simulink model "Logical_Ventilation"  (R2023b)
settings: Solver=VariableStepAuto  StartTime=0.0  StopTime=60  RelTol=1e-3
PostLoadFcn:
  | load data\rel_humidity.mat;
  | load data\rel_humidity_heatedwire.mat;
  | load data\rel_humidityInput.mat;
libraries: slident x2, slpidlib x2
settings Model: DataDictionary=Logical_Ventilation_dict.sldd  Creator=ppatel  LastModifiedBy=ppatel

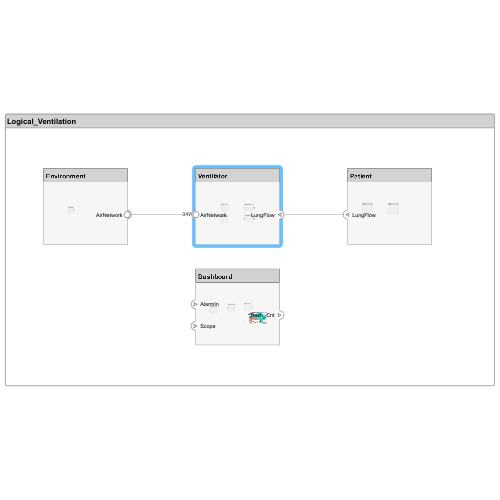
[thumbnail: Simulink's stored preview of the top-level diagram]
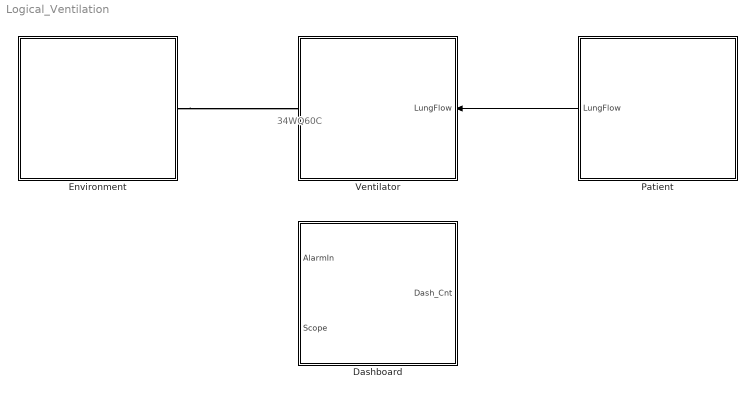
== system Logical_Ventilation ==
  note: 34WQ60C
  Dashboard : Subsystem
      settings: PortSchema="{\"entries\":[{\"content\":{\"headerSize\":26,\"margin\":15,\"minimumSpacing\":25,\"sides\":[{\"content\":{\"connectorIds\":[\"In1\",\"In2\"]},\"type\":\"ConnectorPlacement.EquallySpacedRectSide\",\"uuid\":\"30d5a539-2c7a-40a6-b159-872080309fb0\"},{\"content\":{\"connectorIds\":[\"Out1\"],\"side\":\"RIGHT\"},\"type\":\"ConnectorPlacement.EquallySpacedRectSide\",\"uuid\":\"9c23b845-c6d3-461f-9717-3c81fce4740e\"},{\"content\":{\"side\":\"TOP\"},\"type\":\"ConnectorPlacement.EquallySpacedRectSide\",\"uuid\":\"23e2f61e-2083-47d3-9d3a-aca5cd4f1fc6\"}]},\"type\":\"ConnectorPlacement.EquallySpacedConnector\",\"uuid\":\"a2e9d942-417e-49d1-8834-66036fdf29fe\"}],\"packageUris\":[\"http://schema.mathworks.com/mf0/Connector/R2020b\"],\"version\":\"1.0\"}"
  Environment : Subsystem
      settings: PortSchema="{\"entries\":[{\"content\":{\"headerSize\":26,\"margin\":15,\"minimumSpacing\":25,\"sides\":[{\"content\":{},\"type\":\"ConnectorPlacement.EquallySpacedRectSide\",\"uuid\":\"30d5a539-2c7a-40a6-b159-872080309fb0\"},{\"content\":{\"connectorIds\":[\"RConn1\"],\"side\":\"RIGHT\"},\"type\":\"ConnectorPlacement.EquallySpacedRectSide\",\"uuid\":\"9c23b845-c6d3-461f-9717-3c81fce4740e\"},{\"content\":{\"side\":\"TOP\"},\"type\":\"ConnectorPlacement.EquallySpacedRectSide\",\"uuid\":\"23e2f61e-2083-47d3-9d3a-aca5cd4f1fc6\"}]},\"type\":\"ConnectorPlacement.EquallySpacedConnector\",\"uuid\":\"a2e9d942-417e-49d1-8834-66036fdf29fe\"}],\"packageUris\":[\"http://schema.mathworks.com/mf0/Connector/R2020b\"],\"version\":\"1.0\"}"
  Patient : Subsystem
      settings: PortSchema="{\"entries\":[{\"content\":{\"headerSize\":26,\"margin\":15,\"minimumSpacing\":25,\"sides\":[{\"content\":{\"connectorIds\":[\"Out1\"]},\"type\":\"ConnectorPlacement.EquallySpacedRectSide\",\"uuid\":\"30d5a539-2c7a-40a6-b159-872080309fb0\"},{\"content\":{\"side\":\"RIGHT\"},\"type\":\"ConnectorPlacement.EquallySpacedRectSide\",\"uuid\":\"9c23b845-c6d3-461f-9717-3c81fce4740e\"},{\"content\":{\"side\":\"TOP\"},\"type\":\"ConnectorPlacement.EquallySpacedRectSide\",\"uuid\":\"23e2f61e-2083-47d3-9d3a-aca5cd4f1fc6\"}]},\"type\":\"ConnectorPlacement.EquallySpacedConnector\",\"uuid\":\"a2e9d942-417e-49d1-8834-66036fdf29fe\"}],\"packageUris\":[\"http://schema.mathworks.com/mf0/Connector/R2020b\"],\"version\":\"1.0\"}"
  Ventilator : Subsystem
      settings: PortSchema="{\"entries\":[{\"content\":{\"headerSize\":26,\"margin\":15,\"minimumSpacing\":25,\"sides\":[{\"content\":{\"connectorIds\":[\"RConn1\"]},\"type\":\"ConnectorPlacement.EquallySpacedRectSide\",\"uuid\":\"30d5a539-2c7a-40a6-b159-872080309fb0\"},{\"content\":{\"connectorIds\":[\"In1\"],\"side\":\"RIGHT\"},\"type\":\"ConnectorPlacement.EquallySpacedRectSide\",\"uuid\":\"9c23b845-c6d3-461f-9717-3c81fce4740e\"},{\"content\":{\"side\":\"TOP\"},\"type\":\"ConnectorPlacement.EquallySpacedRectSide\",\"uuid\":\"23e2f61e-2083-47d3-9d3a-aca5cd4f1fc6\"}]},\"type\":\"ConnectorPlacement.EquallySpacedConnector\",\"uuid\":\"a2e9d942-417e-49d1-8834-66036fdf29fe\"}],\"packageUris\":[\"http://schema.mathworks.com/mf0/Connector/R2020b\"],\"version\":\"1.0\"}"
  wires:
  Patient/1(LungFlow) -> Ventilator/1(LungFlow)
  connections:
  Environment/RConn1 -- Ventilator/RConn1

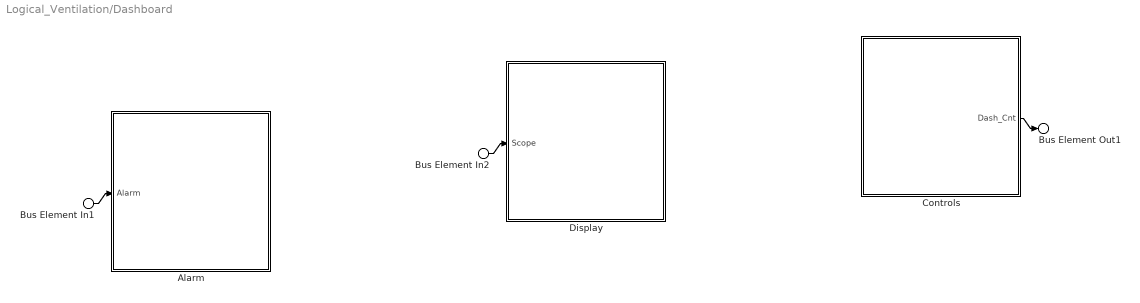
== system Logical_Ventilation/Dashboard ==
  Bus Element In1 : Inport  PortName=AlarmIn
  Bus Element In2 : Inport  Port=2  PortName=Scope
  Alarm : Subsystem
      settings: PortSchema="{\"entries\":[{\"content\":{\"headerSize\":26,\"margin\":15,\"minimumSpacing\":25,\"sides\":[{\"content\":{\"connectorIds\":[\"In1\"]},\"type\":\"ConnectorPlacement.EquallySpacedRectSide\",\"uuid\":\"30d5a539-2c7a-40a6-b159-872080309fb0\"},{\"content\":{\"side\":\"RIGHT\"},\"type\":\"ConnectorPlacement.EquallySpacedRectSide\",\"uuid\":\"9c23b845-c6d3-461f-9717-3c81fce4740e\"},{\"content\":{\"side\":\"TOP\"},\"type\":\"ConnectorPlacement.EquallySpacedRectSide\",\"uuid\":\"23e2f61e-2083-47d3-9d3a-aca5cd4f1fc6\"}]},\"type\":\"ConnectorPlacement.EquallySpacedConnector\",\"uuid\":\"a2e9d942-417e-49d1-8834-66036fdf29fe\"}],\"packageUris\":[\"http://schema.mathworks.com/mf0/Connector/R2020b\"],\"version\":\"1.0\"}"
  Controls : Subsystem
      settings: PortSchema="{\"entries\":[{\"content\":{\"headerSize\":26,\"margin\":15,\"minimumSpacing\":25,\"sides\":[{\"content\":{},\"type\":\"ConnectorPlacement.EquallySpacedRectSide\",\"uuid\":\"30d5a539-2c7a-40a6-b159-872080309fb0\"},{\"content\":{\"connectorIds\":[\"Out1\"],\"side\":\"RIGHT\"},\"type\":\"ConnectorPlacement.EquallySpacedRectSide\",\"uuid\":\"9c23b845-c6d3-461f-9717-3c81fce4740e\"},{\"content\":{\"side\":\"TOP\"},\"type\":\"ConnectorPlacement.EquallySpacedRectSide\",\"uuid\":\"23e2f61e-2083-47d3-9d3a-aca5cd4f1fc6\"}]},\"type\":\"ConnectorPlacement.EquallySpacedConnector\",\"uuid\":\"a2e9d942-417e-49d1-8834-66036fdf29fe\"}],\"packageUris\":[\"http://schema.mathworks.com/mf0/Connector/R2020b\"],\"version\":\"1.0\"}"
  Display : Subsystem
      settings: PortSchema="{\"entries\":[{\"content\":{\"headerSize\":26,\"margin\":15,\"minimumSpacing\":25,\"sides\":[{\"content\":{\"connectorIds\":[\"In1\"]},\"type\":\"ConnectorPlacement.EquallySpacedRectSide\",\"uuid\":\"30d5a539-2c7a-40a6-b159-872080309fb0\"},{\"content\":{\"side\":\"RIGHT\"},\"type\":\"ConnectorPlacement.EquallySpacedRectSide\",\"uuid\":\"9c23b845-c6d3-461f-9717-3c81fce4740e\"},{\"content\":{\"side\":\"TOP\"},\"type\":\"ConnectorPlacement.EquallySpacedRectSide\",\"uuid\":\"23e2f61e-2083-47d3-9d3a-aca5cd4f1fc6\"}]},\"type\":\"ConnectorPlacement.EquallySpacedConnector\",\"uuid\":\"a2e9d942-417e-49d1-8834-66036fdf29fe\"}],\"packageUris\":[\"http://schema.mathworks.com/mf0/Connector/R2020b\"],\"version\":\"1.0\"}"
  Bus Element Out1 : Outport  PortName=Dash_Cnt
  wires:
  Controls/1(Dash_Cnt) -> Bus Element Out1/1
  Bus Element In2/1 -> Display/1(Scope)
  Bus Element In1/1 -> Alarm/1(Alarm)

== system Logical_Ventilation/Environment ==
  Source_Sink_Air : Subsystem
      settings: PortSchema="{\"entries\":[{\"content\":{\"headerSize\":26,\"margin\":15,\"minimumSpacing\":25,\"sides\":[{\"content\":{},\"type\":\"ConnectorPlacement.EquallySpacedRectSide\",\"uuid\":\"30d5a539-2c7a-40a6-b159-872080309fb0\"},{\"content\":{\"connectorIds\":[\"RConn1\"],\"side\":\"RIGHT\"},\"type\":\"ConnectorPlacement.EquallySpacedRectSide\",\"uuid\":\"9c23b845-c6d3-461f-9717-3c81fce4740e\"},{\"content\":{\"side\":\"TOP\"},\"type\":\"ConnectorPlacement.EquallySpacedRectSide\",\"uuid\":\"23e2f61e-2083-47d3-9d3a-aca5cd4f1fc6\"}]},\"type\":\"ConnectorPlacement.EquallySpacedConnector\",\"uuid\":\"a2e9d942-417e-49d1-8834-66036fdf29fe\"}],\"packageUris\":[\"http://schema.mathworks.com/mf0/Connector/R2020b\"],\"version\":\"1.0\"}"
  AirNetwork : PMIOPort  Side=Right  ConnectionType=Bus: AirSupply
  connections:
  Source_Sink_Air/RConn1 -- AirNetwork/RConn1

== system Logical_Ventilation/Patient ==
  Lung : Subsystem
      settings: PortSchema="{\"entries\":[{\"content\":{\"headerSize\":26,\"margin\":15,\"minimumSpacing\":25,\"sides\":[{\"content\":{},\"type\":\"ConnectorPlacement.EquallySpacedRectSide\",\"uuid\":\"30d5a539-2c7a-40a6-b159-872080309fb0\"},{\"content\":{\"side\":\"RIGHT\"},\"type\":\"ConnectorPlacement.EquallySpacedRectSide\",\"uuid\":\"9c23b845-c6d3-461f-9717-3c81fce4740e\"},{\"content\":{\"side\":\"TOP\"},\"type\":\"ConnectorPlacement.EquallySpacedRectSide\",\"uuid\":\"23e2f61e-2083-47d3-9d3a-aca5cd4f1fc6\"}]},\"type\":\"ConnectorPlacement.EquallySpacedConnector\",\"uuid\":\"a2e9d942-417e-49d1-8834-66036fdf29fe\"}],\"packageUris\":[\"http://schema.mathworks.com/mf0/Connector/R2020b\"],\"version\":\"1.0\"}"
  Mask : Subsystem
      settings: PortSchema="{\"entries\":[{\"content\":{\"headerSize\":26,\"margin\":15,\"minimumSpacing\":25,\"sides\":[{\"content\":{},\"type\":\"ConnectorPlacement.EquallySpacedRectSide\",\"uuid\":\"30d5a539-2c7a-40a6-b159-872080309fb0\"},{\"content\":{\"side\":\"RIGHT\"},\"type\":\"ConnectorPlacement.EquallySpacedRectSide\",\"uuid\":\"9c23b845-c6d3-461f-9717-3c81fce4740e\"},{\"content\":{\"side\":\"TOP\"},\"type\":\"ConnectorPlacement.EquallySpacedRectSide\",\"uuid\":\"23e2f61e-2083-47d3-9d3a-aca5cd4f1fc6\"}]},\"type\":\"ConnectorPlacement.EquallySpacedConnector\",\"uuid\":\"a2e9d942-417e-49d1-8834-66036fdf29fe\"}],\"packageUris\":[\"http://schema.mathworks.com/mf0/Connector/R2020b\"],\"version\":\"1.0\"}"
  Bus Element Out1 : Outport  PortName=LungFlow

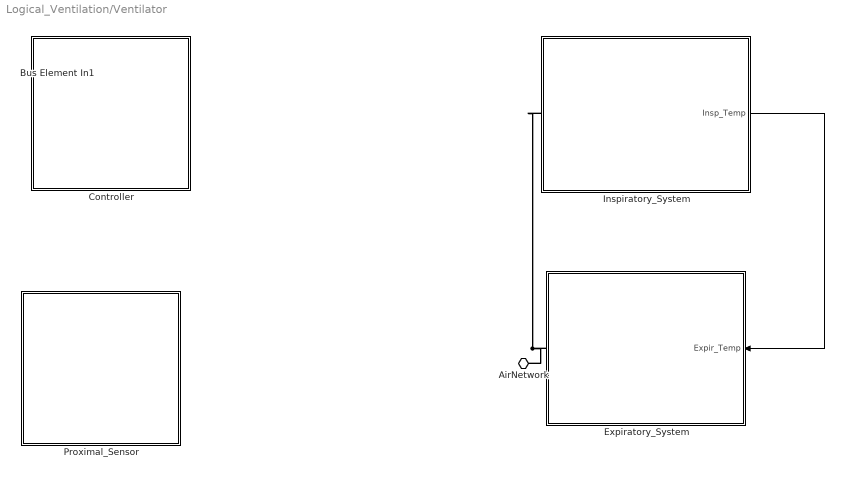
== system Logical_Ventilation/Ventilator ==
  Bus Element In1 : Inport  PortName=LungFlow
  Controller : Subsystem
      settings: PortSchema="{\"entries\":[{\"content\":{\"headerSize\":26,\"margin\":15,\"minimumSpacing\":25,\"sides\":[{\"content\":{},\"type\":\"ConnectorPlacement.EquallySpacedRectSide\",\"uuid\":\"30d5a539-2c7a-40a6-b159-872080309fb0\"},{\"content\":{\"side\":\"RIGHT\"},\"type\":\"ConnectorPlacement.EquallySpacedRectSide\",\"uuid\":\"9c23b845-c6d3-461f-9717-3c81fce4740e\"},{\"content\":{\"side\":\"TOP\"},\"type\":\"ConnectorPlacement.EquallySpacedRectSide\",\"uuid\":\"23e2f61e-2083-47d3-9d3a-aca5cd4f1fc6\"}]},\"type\":\"ConnectorPlacement.EquallySpacedConnector\",\"uuid\":\"a2e9d942-417e-49d1-8834-66036fdf29fe\"}],\"packageUris\":[\"http://schema.mathworks.com/mf0/Connector/R2020b\"],\"version\":\"1.0\"}"
  Expiratory_System : Subsystem
      settings: PortSchema="{\"entries\":[{\"content\":{\"headerSize\":26,\"margin\":15,\"minimumSpacing\":25,\"sides\":[{\"content\":{\"connectorIds\":[\"LConn1\"]},\"type\":\"ConnectorPlacement.EquallySpacedRectSide\",\"uuid\":\"30d5a539-2c7a-40a6-b159-872080309fb0\"},{\"content\":{\"connectorIds\":[\"In1\"],\"side\":\"RIGHT\"},\"type\":\"ConnectorPlacement.EquallySpacedRectSide\",\"uuid\":\"9c23b845-c6d3-461f-9717-3c81fce4740e\"},{\"content\":{\"side\":\"TOP\"},\"type\":\"ConnectorPlacement.EquallySpacedRectSide\",\"uuid\":\"23e2f61e-2083-47d3-9d3a-aca5cd4f1fc6\"}]},\"type\":\"ConnectorPlacement.EquallySpacedConnector\",\"uuid\":\"a2e9d942-417e-49d1-8834-66036fdf29fe\"}],\"packageUris\":[\"http://schema.mathworks.com/mf0/Connector/R2020b\"],\"version\":\"1.0\"}"
  Inspiratory_System : Subsystem
      settings: PortSchema="{\"entries\":[{\"content\":{\"headerSize\":26,\"margin\":15,\"minimumSpacing\":25,\"sides\":[{\"content\":{\"connectorIds\":[\"LConn1\"]},\"type\":\"ConnectorPlacement.EquallySpacedRectSide\",\"uuid\":\"30d5a539-2c7a-40a6-b159-872080309fb0\"},{\"content\":{\"connectorIds\":[\"Out1\"],\"side\":\"RIGHT\"},\"type\":\"ConnectorPlacement.EquallySpacedRectSide\",\"uuid\":\"9c23b845-c6d3-461f-9717-3c81fce4740e\"},{\"content\":{\"side\":\"TOP\"},\"type\":\"ConnectorPlacement.EquallySpacedRectSide\",\"uuid\":\"23e2f61e-2083-47d3-9d3a-aca5cd4f1fc6\"}]},\"type\":\"ConnectorPlacement.EquallySpacedConnector\",\"uuid\":\"a2e9d942-417e-49d1-8834-66036fdf29fe\"}],\"packageUris\":[\"http://schema.mathworks.com/mf0/Connector/R2020b\"],\"version\":\"1.0\"}"
  Proximal_Sensor : Subsystem
      settings: PortSchema="{\"entries\":[{\"content\":{\"headerSize\":26,\"margin\":15,\"minimumSpacing\":25,\"sides\":[{\"content\":{},\"type\":\"ConnectorPlacement.EquallySpacedRectSide\",\"uuid\":\"30d5a539-2c7a-40a6-b159-872080309fb0\"},{\"content\":{\"side\":\"RIGHT\"},\"type\":\"ConnectorPlacement.EquallySpacedRectSide\",\"uuid\":\"9c23b845-c6d3-461f-9717-3c81fce4740e\"},{\"content\":{\"side\":\"TOP\"},\"type\":\"ConnectorPlacement.EquallySpacedRectSide\",\"uuid\":\"23e2f61e-2083-47d3-9d3a-aca5cd4f1fc6\"}]},\"type\":\"ConnectorPlacement.EquallySpacedConnector\",\"uuid\":\"a2e9d942-417e-49d1-8834-66036fdf29fe\"}],\"packageUris\":[\"http://schema.mathworks.com/mf0/Connector/R2020b\"],\"version\":\"1.0\"}"
  AirNetwork : PMIOPort  Side=Right  ConnectionType=Bus: AirSupply
  wires:
  Inspiratory_System/1(Insp_Temp) -> Expiratory_System/1(Expir_Temp)
  connections:
  Inspiratory_System/LConn1 -- Expiratory_System/LConn1 -- AirNetwork/RConn1

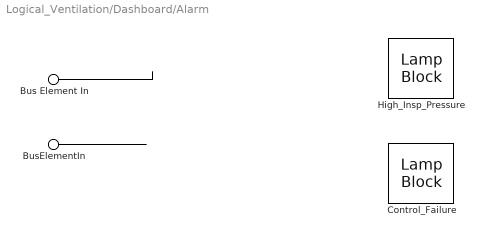
== system Logical_Ventilation/Dashboard/Alarm ==
  Bus Element In : Inport  PortName=Alarm  Element=HPress
  BusElementIn : Inport  PortName=Alarm  Element=CFail
  Control_Failure : LampBlock  LabelPosition=Hide
  High_Insp_Pressure : LampBlock  LabelPosition=Hide
  wires:
  Bus Element In/1 -> ?
  BusElementIn/1 -> ?

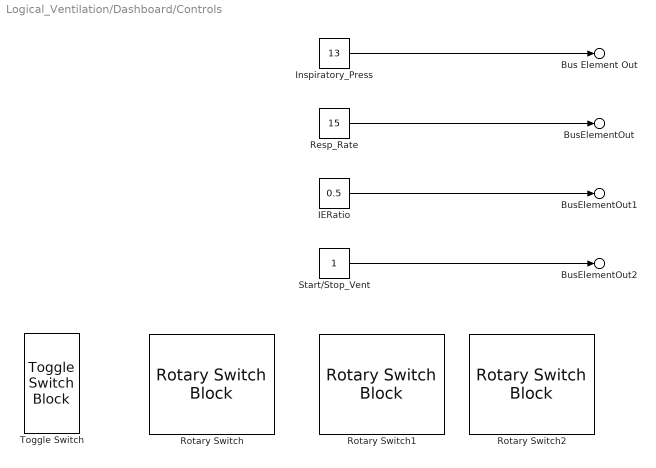
== system Logical_Ventilation/Dashboard/Controls ==
  IERatio : Constant  Value=0.5
  Inspiratory_Press : Constant  Value=13  OutDataTypeStr=uint8
  Resp_Rate : Constant  Value=15  OutDataTypeStr=uint8
  Rotary Switch : RotarySwitchBlock
      settings: Values={{'Off', 'Low', 'Medium', 'High'}, [5 13 22 26]}
  Rotary Switch1 : RotarySwitchBlock
      settings: Values={{'5', '10', '15', '20', '25'}, [5 10 15 20 25]}
  Rotary Switch2 : RotarySwitchBlock
      settings: Values={{'1:3', '1:2', '1:1', '2:1'}, [0.33 0.5 1 2]}
  Start/Stop_Vent : Constant  OutDataTypeStr=boolean
  Toggle Switch : ToggleSwitchBlock
      settings: Values={{'Stop', 'Start'}, [0 1]}
  Bus Element Out : Outport  PortName=Dash_Cnt  Element=insp_press
  BusElementOut : Outport  PortName=Dash_Cnt  Element=RR
  BusElementOut1 : Outport  PortName=Dash_Cnt  Element=IERatio
  BusElementOut2 : Outport  PortName=Dash_Cnt  Element=StartStopVent
  wires:
  Resp_Rate/1 -> BusElementOut/1
  IERatio/1 -> BusElementOut1/1
  Inspiratory_Press/1 -> Bus Element Out/1
  Start/Stop_Vent/1 -> BusElementOut2/1

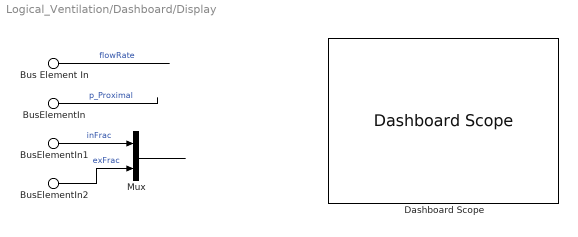
== system Logical_Ventilation/Dashboard/Display ==
  Bus Element In : Inport  PortName=Scope  Element=flowRate
  BusElementIn : Inport  PortName=Scope  Element=pProximal
  BusElementIn1 : Inport  PortName=Scope  Element=inValveFrac
  BusElementIn2 : Inport  PortName=Scope  Element=exValve
  Dashboard Scope : DashboardScope
  Mux : Mux  Inputs=2
  wires:
  Bus Element In/1 -> ?  "flowRate"
  BusElementIn1/1 -> Mux/1  "inFrac"
  BusElementIn2/1 -> Mux/2  "exFrac"
  Mux/1 -> ?
  BusElementIn/1 -> ?  "p_Proximal"

== system Logical_Ventilation/Environment/Source_Sink_Air ==
  AirNetwork : PMIOPort  Side=Right

== system Logical_Ventilation/Patient/Lung ==

== system Logical_Ventilation/Patient/Mask ==

== system Logical_Ventilation/Ventilator/Controller ==

== system Logical_Ventilation/Ventilator/Expiratory_System ==
  Bus Element In1 : Inport  PortName=Expir_Temp
  Expiratory_Tube : Subsystem
      settings: PortSchema="{\"entries\":[{\"content\":{\"headerSize\":26,\"margin\":15,\"minimumSpacing\":25,\"sides\":[{\"content\":{},\"type\":\"ConnectorPlacement.EquallySpacedRectSide\",\"uuid\":\"30d5a539-2c7a-40a6-b159-872080309fb0\"},{\"content\":{\"connectorIds\":[\"In1\"],\"side\":\"RIGHT\"},\"type\":\"ConnectorPlacement.EquallySpacedRectSide\",\"uuid\":\"9c23b845-c6d3-461f-9717-3c81fce4740e\"},{\"content\":{\"side\":\"TOP\"},\"type\":\"ConnectorPlacement.EquallySpacedRectSide\",\"uuid\":\"23e2f61e-2083-47d3-9d3a-aca5cd4f1fc6\"}]},\"type\":\"ConnectorPlacement.EquallySpacedConnector\",\"uuid\":\"a2e9d942-417e-49d1-8834-66036fdf29fe\"}],\"packageUris\":[\"http://schema.mathworks.com/mf0/Connector/R2020b\"],\"version\":\"1.0\"}"
  CO2Delivery : PMIOPort  Side=Left
  wires:
  Bus Element In1/1 -> Expiratory_Tube/1(ExpirTube_Temp)

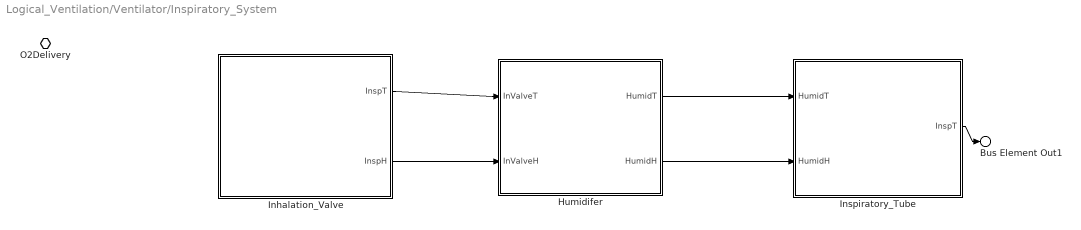
== system Logical_Ventilation/Ventilator/Inspiratory_System ==
  Humidifer : Subsystem
      settings: PortSchema="{\"entries\":[{\"content\":{\"headerSize\":26,\"margin\":15,\"minimumSpacing\":25,\"sides\":[{\"content\":{\"connectorIds\":[\"In1\",\"In2\"]},\"type\":\"ConnectorPlacement.EquallySpacedRectSide\",\"uuid\":\"30d5a539-2c7a-40a6-b159-872080309fb0\"},{\"content\":{\"connectorIds\":[\"Out2\",\"Out1\"],\"side\":\"RIGHT\"},\"type\":\"ConnectorPlacement.EquallySpacedRectSide\",\"uuid\":\"9c23b845-c6d3-461f-9717-3c81fce4740e\"},{\"content\":{\"side\":\"TOP\"},\"type\":\"ConnectorPlacement.EquallySpacedRectSide\",\"uuid\":\"23e2f61e-2083-47d3-9d3a-aca5cd4f1fc6\"}]},\"type\":\"ConnectorPlacement.EquallySpacedConnector\",\"uuid\":\"a2e9d942-417e-49d1-8834-66036fdf29fe\"}],\"packageUris\":[\"http://schema.mathworks.com/mf0/Connector/R2020b\"],\"version\":\"1.0\"}"
  Inhalation_Valve : Subsystem
      settings: PortSchema="{\"entries\":[{\"content\":{\"headerSize\":26,\"margin\":15,\"minimumSpacing\":25,\"sides\":[{\"content\":{},\"type\":\"ConnectorPlacement.EquallySpacedRectSide\",\"uuid\":\"30d5a539-2c7a-40a6-b159-872080309fb0\"},{\"content\":{\"connectorIds\":[\"Out1\",\"Out2\"],\"side\":\"RIGHT\"},\"type\":\"ConnectorPlacement.EquallySpacedRectSide\",\"uuid\":\"9c23b845-c6d3-461f-9717-3c81fce4740e\"},{\"content\":{\"side\":\"TOP\"},\"type\":\"ConnectorPlacement.EquallySpacedRectSide\",\"uuid\":\"23e2f61e-2083-47d3-9d3a-aca5cd4f1fc6\"}]},\"type\":\"ConnectorPlacement.EquallySpacedConnector\",\"uuid\":\"a2e9d942-417e-49d1-8834-66036fdf29fe\"}],\"packageUris\":[\"http://schema.mathworks.com/mf0/Connector/R2020b\"],\"version\":\"1.0\"}"
  Inspiratory_Tube : Subsystem
      settings: PortSchema="{\"entries\":[{\"content\":{\"headerSize\":26,\"margin\":15,\"minimumSpacing\":25,\"sides\":[{\"content\":{\"connectorIds\":[\"In2\",\"In1\"]},\"type\":\"ConnectorPlacement.EquallySpacedRectSide\",\"uuid\":\"30d5a539-2c7a-40a6-b159-872080309fb0\"},{\"content\":{\"connectorIds\":[\"Out1\"],\"side\":\"RIGHT\"},\"type\":\"ConnectorPlacement.EquallySpacedRectSide\",\"uuid\":\"9c23b845-c6d3-461f-9717-3c81fce4740e\"},{\"content\":{\"side\":\"TOP\"},\"type\":\"ConnectorPlacement.EquallySpacedRectSide\",\"uuid\":\"23e2f61e-2083-47d3-9d3a-aca5cd4f1fc6\"}]},\"type\":\"ConnectorPlacement.EquallySpacedConnector\",\"uuid\":\"a2e9d942-417e-49d1-8834-66036fdf29fe\"}],\"packageUris\":[\"http://schema.mathworks.com/mf0/Connector/R2020b\"],\"version\":\"1.0\"}"
  O2Delivery : PMIOPort  Side=Left
  Bus Element Out1 : Outport  PortName=Insp_Temp
  wires:
  Inhalation_Valve/1(InspT) -> Humidifer/1(InValveT)
  Inhalation_Valve/2(InspH) -> Humidifer/2(InValveH)
  Humidifer/1(HumidH) -> Inspiratory_Tube/1(HumidH)
  Humidifer/2(HumidT) -> Inspiratory_Tube/2(HumidT)
  Inspiratory_Tube/1(InspT) -> Bus Element Out1/1

== system Logical_Ventilation/Ventilator/Proximal_Sensor ==

== system Logical_Ventilation/Ventilator/Expiratory_System/Expiratory_Tube ==
  Bus Element In1 : Inport  PortName=ExpirTube_Temp
  CheckValve : Subsystem
      settings: PortSchema="{\"entries\":[{\"content\":{\"headerSize\":26,\"margin\":15,\"minimumSpacing\":25,\"sides\":[{\"content\":{},\"type\":\"ConnectorPlacement.EquallySpacedRectSide\",\"uuid\":\"30d5a539-2c7a-40a6-b159-872080309fb0\"},{\"content\":{\"side\":\"RIGHT\"},\"type\":\"ConnectorPlacement.EquallySpacedRectSide\",\"uuid\":\"9c23b845-c6d3-461f-9717-3c81fce4740e\"},{\"content\":{\"side\":\"TOP\"},\"type\":\"ConnectorPlacement.EquallySpacedRectSide\",\"uuid\":\"23e2f61e-2083-47d3-9d3a-aca5cd4f1fc6\"}]},\"type\":\"ConnectorPlacement.EquallySpacedConnector\",\"uuid\":\"a2e9d942-417e-49d1-8834-66036fdf29fe\"}],\"packageUris\":[\"http://schema.mathworks.com/mf0/Connector/R2020b\"],\"version\":\"1.0\"}"
  Temp_RH_Sensor : Subsystem
      settings: PortSchema="{\"entries\":[{\"content\":{\"headerSize\":26,\"margin\":15,\"minimumSpacing\":25,\"sides\":[{\"content\":{},\"type\":\"ConnectorPlacement.EquallySpacedRectSide\",\"uuid\":\"30d5a539-2c7a-40a6-b159-872080309fb0\"},{\"content\":{\"connectorIds\":[\"In1\"],\"side\":\"RIGHT\"},\"type\":\"ConnectorPlacement.EquallySpacedRectSide\",\"uuid\":\"9c23b845-c6d3-461f-9717-3c81fce4740e\"},{\"content\":{\"side\":\"TOP\"},\"type\":\"ConnectorPlacement.EquallySpacedRectSide\",\"uuid\":\"23e2f61e-2083-47d3-9d3a-aca5cd4f1fc6\"}]},\"type\":\"ConnectorPlacement.EquallySpacedConnector\",\"uuid\":\"a2e9d942-417e-49d1-8834-66036fdf29fe\"}],\"packageUris\":[\"http://schema.mathworks.com/mf0/Connector/R2020b\"],\"version\":\"1.0\"}"
  wires:
  Bus Element In1/1 -> Temp_RH_Sensor/1(ExpSens_T)

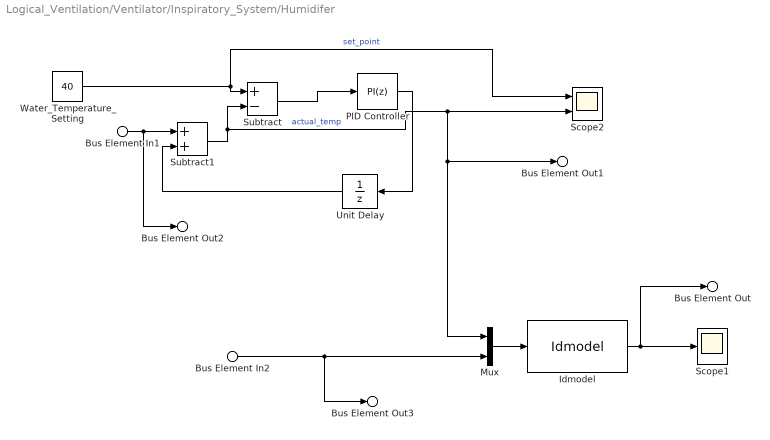
== system Logical_Ventilation/Ventilator/Inspiratory_System/Humidifer ==
  Bus Element In1 : Inport  PortName=InValveT  Element=Room_T
  Bus Element In2 : Inport  Port=2  PortName=InValveH  Element=Room_H
  Idmodel : slident/Models/Idmodel  sys=mp  IC=0  noi=on  seed=[]
  Mux : Mux  Inputs=2
  PID Controller : slpidlib/PID Controller  Controller=PI  Form=Parallel  TimeDomain=Discrete-time  UseExternalTs=off  SampleTime=0.05  IntegratorMethod=Forward Euler  FilterMethod=Forward Euler  ControllerParametersSource=internal  P=0.0103828718955391  I=0.415314875821562  UseKiTs=off  D=0  N=100  UseFilter=on  TunerSelectOption=Transfer Function Based (PID Tuner App)  InitialConditionSource=internal  InitialConditionForIntegrator=0  InitialConditionForFilter=0  DifferentiatorICPrevScaledInput=0  ExternalReset=none  TrackingMode=off  Kt=1  LimitOutput=off  SatLimitsSource=internal  UpperSaturationLimit=inf  LowerSaturationLimit=-inf  LinearizeAsGain=on  AntiWindupMode=none  Kb=1  LimitIntegrator=off  UpperIntegratorSaturationLimit=inf  LowerIntegratorSaturationLimit=-inf  POutMin=[]  POutMax=[]  IOutMin=[]  IOutMax=[]  DOutMin=[]  DOutMax=[]  NOutMin=[]  NOutMax=[]  SumOutMin=[]  SumOutMax=[]  SaturationOutMin=[]  SaturationOutMax=[]  PParamMin=[]  PParamMax=[]  IParamMin=[]  IParamMax=[]  DParamMin=[]  DParamMax=[]  NParamMin=[]  NParamMax=[]  KbParamMin=[]  KbParamMax=[]  KtParamMin=[]  KtParamMax=[]  KbOutMin=[]  KbOutMax=[]  KtOutMin=[]  KtOutMax=[]  IntegratorOutMin=[]  IntegratorOutMax=[]  FilterOutMin=[]  FilterOutMax=[]  SumI1OutMin=[]  SumI1OutMax=[]  SumI2OutMin=[]  SumI2OutMax=[]  SumI3OutMin=[]  SumI3OutMax=[]  SumI4OutMin=[]  SumI4OutMax=[]  SumDOutMin=[]  SumDOutMax=[]  DifferentiatorOutMin=[]  DifferentiatorOutMax=[]  FilterDiffOutCoefMin=[]  FilterDiffOutCoefMax=[]  ReciprocalOutMin=[]  ReciprocalOutMax=[]  SumDenOutMin=[]  SumDenOutMax=[]  SumNumOutMin=[]  SumNumOutMax=[]  DivideOutMin=[]  DivideOutMax=[]  UdiffTsProdOutMin=[]  UdiffTsProdOutMax=[]  NTsProdOutMin=[]  NTsProdOutMax=[]  UintegralTsProdOutMin=[]  UintegralTsProdOutMax=[]  UngainTsProdOutMin=[]  UngainTsProdOutMax=[]  ClampingZeroOutDataTypeStr=Inherit: Inherit via back propagation  ClampingZeroOutMin=[]  ClampingZeroOutMax=[]  FilterDenConstantOutDataTypeStr=Inherit: Inherit via back propagation  FilterDenConstantOutMin=[]  FilterDenConstantOutMax=[]  PCopyOutDataTypeStr=Inherit: Inherit via back propagation  PCopyOutMin=[]  PCopyOutMax=[]  NCopyOutDataTypeStr=Inherit: Inherit via back propagation  NCopyOutMin=[]  NCopyOutMax=[]  IntegratorContinuousStateAttributes=''  IntegratorStateMustResolveToSignalObject=off  IntegratorRTWStateStorageClass=Auto  FilterContinuousStateAttributes=''  FilterStateMustResolveToSignalObject=off  FilterRTWStateStorageClass=Auto  ParallelPVariant=InternalParameters  IdealPVariant=Disabled  IVariant=InternalParameters  DVariant=Disabled  IntegratorVariant=Discrete  SatVariant=Disabled  AWVariant=Passthrough  PCopyVariant=Disabled  TRVariant=Disabled  FdbkBlocksVariant=Forward  IdealPFdbkVariant=Disabled  SatFdbkVariant=Disabled  DerivativeFilterVariant=Disabled  NVariant=Disabled  NCopyVariant=Disabled_SignalSpec  FilterICVariant=Disabled  IntegratorICVariant=InternalICs  ExternalResetVariant=Disabled  TRSumVariant=Passthrough  SumFdbkVariant=Disabled  SumVariant=Sum_PI  TsampFilterVariant=InternalTs  TsampNgainVariant=Passthrough  TsampIntegralVariant=Disabled_SignalSpec  ExternalSaturationOutDataTypeStr=Inherit: Same as second input
  Scope1 : Scope
  Scope2 : Scope  NumInputPorts=2
  Subtract : Sum  Inputs=+-
  Subtract1 : Sum
  Unit Delay : UnitDelay  SampleTime=-1  HasFrameUpgradeWarning=on
  Water_Temperature_Setting : Constant  Value=40
  Bus Element Out3 : Outport  PortName=HumidH  Element=Room_H
  Bus Element Out : Outport  PortName=HumidH  Element=Humidifier_H
  Bus Element Out2 : Outport  Port=2  PortName=HumidT  Element=Room_T
  Bus Element Out1 : Outport  Port=2  PortName=HumidT  Element=Water_T
  wires:
  Unit Delay/1 -> Subtract1/2
  Water_Temperature_Setting/1 -> Scope2/1, Subtract/1  "set_point"
  Subtract1/1 -> Bus Element Out1/1, Mux/1, Scope2/2, Subtract/2  "actual_temp"
  PID Controller/1 -> Unit Delay/1
  Subtract/1 -> PID Controller/1
  Bus Element In2/1 -> Bus Element Out3/1, Mux/2
  Mux/1 -> Idmodel/1
  Idmodel/1 -> Bus Element Out/1, Scope1/1
  Bus Element In1/1 -> Bus Element Out2/1, Subtract1/1

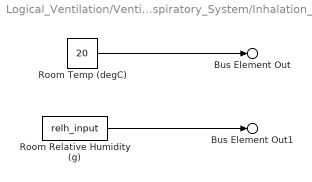
== system Logical_Ventilation/Ventilator/Inspiratory_System/Inhalation_Valve ==
  Room Relative Humidity (g) : FromWorkspace  VariableName=relh_input  OutDataTypeStr=double
  Room Temp (degC) : Constant  Value=20
  Bus Element Out : Outport  PortName=InspT  Element=Room_T
  Bus Element Out1 : Outport  Port=2  PortName=InspH  Element=Room_H
  wires:
  Room Temp (degC)/1 -> Bus Element Out/1
  Room Relative Humidity (g)/1 -> Bus Element Out1/1

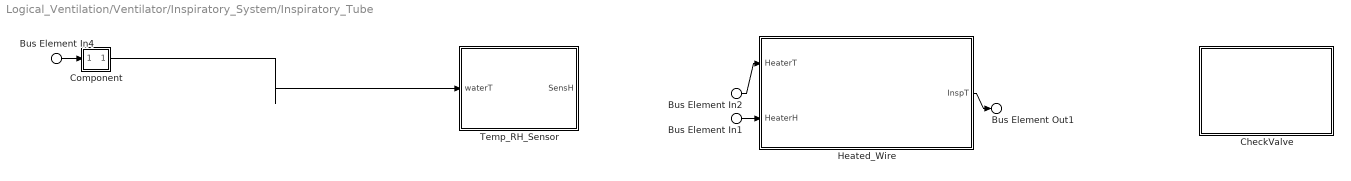
== system Logical_Ventilation/Ventilator/Inspiratory_System/Inspiratory_Tube ==
  Bus Element In1 : Inport  PortName=HumidH
  Bus Element In2 : Inport  Port=2  PortName=HumidT
  Bus Element In4 : Inport  Port=2  PortName=HumidT
  CheckValve : Subsystem
      settings: PortSchema="{\"entries\":[{\"content\":{\"headerSize\":26,\"margin\":15,\"minimumSpacing\":25,\"sides\":[{\"content\":{},\"type\":\"ConnectorPlacement.EquallySpacedRectSide\",\"uuid\":\"c28154e5-eaf5-480f-8066-17b2d40a2bdd\"},{\"content\":{\"side\":\"RIGHT\"},\"type\":\"ConnectorPlacement.EquallySpacedRectSide\",\"uuid\":\"c3e70359-248e-4787-971d-b6b9bea98e42\"},{\"content\":{\"side\":\"TOP\"},\"type\":\"ConnectorPlacement.EquallySpacedRectSide\",\"uuid\":\"d2a5be48-e58c-43bd-a458-b63b8b525dc1\"}]},\"type\":\"ConnectorPlacement.EquallySpacedConnector\",\"uuid\":\"4afb880b-0c9a-4048-831b-5d1f8f54d79c\"}],\"packageUris\":[\"http://schema.mathworks.com/mf0/Connector/R2020b\"],\"version\":\"1.0\"}"
  Component : Subsystem
      settings: PortSchema="{\"entries\":[{\"content\":{\"margin\":10,\"minimumSpacing\":15,\"sides\":[{\"content\":{\"connectorIds\":[\"In1\"]},\"type\":\"ConnectorPlacement.EquallySpacedRectSide\",\"uuid\":\"ad8c2344-4809-4832-ae62-0542e39a6856\"},{\"content\":{\"connectorIds\":[\"Out1\"],\"side\":\"RIGHT\"},\"type\":\"ConnectorPlacement.EquallySpacedRectSide\",\"uuid\":\"33082802-14bb-48ab-8efd-54a486fc0ece\"},{\"content\":{\"side\":\"TOP\"},\"type\":\"ConnectorPlacement.EquallySpacedRectSide\",\"uuid\":\"4e03c195-d332-43d0-aeb9-c5e6eda740ab\"}]},\"type\":\"ConnectorPlacement.EquallySpacedConnector\",\"uuid\":\"d0446147-b41e-4bb8-8f56-ac2a90a5b24d\"}],\"packageUris\":[\"http://schema.mathworks.com/mf0/Connector/R2020b\"],\"version\":\"1.0\"}"
  Heated_Wire : Subsystem
      settings: PortSchema="{\"entries\":[{\"content\":{\"headerSize\":26,\"margin\":15,\"minimumSpacing\":25,\"sides\":[{\"content\":{\"connectorIds\":[\"In1\",\"In2\"]},\"type\":\"ConnectorPlacement.EquallySpacedRectSide\",\"uuid\":\"c28154e5-eaf5-480f-8066-17b2d40a2bdd\"},{\"content\":{\"connectorIds\":[\"Out1\"],\"side\":\"RIGHT\"},\"type\":\"ConnectorPlacement.EquallySpacedRectSide\",\"uuid\":\"c3e70359-248e-4787-971d-b6b9bea98e42\"},{\"content\":{\"side\":\"TOP\"},\"type\":\"ConnectorPlacement.EquallySpacedRectSide\",\"uuid\":\"d2a5be48-e58c-43bd-a458-b63b8b525dc1\"}]},\"type\":\"ConnectorPlacement.EquallySpacedConnector\",\"uuid\":\"4afb880b-0c9a-4048-831b-5d1f8f54d79c\"}],\"packageUris\":[\"http://schema.mathworks.com/mf0/Connector/R2020b\"],\"version\":\"1.0\"}"
  Temp_RH_Sensor : Subsystem
      settings: PortSchema="{\"entries\":[{\"content\":{\"headerSize\":26,\"margin\":15,\"minimumSpacing\":25,\"sides\":[{\"content\":{\"connectorIds\":[\"In1\"]},\"type\":\"ConnectorPlacement.EquallySpacedRectSide\",\"uuid\":\"30d5a539-2c7a-40a6-b159-872080309fb0\"},{\"content\":{\"connectorIds\":[\"Out1\"],\"side\":\"RIGHT\"},\"type\":\"ConnectorPlacement.EquallySpacedRectSide\",\"uuid\":\"9c23b845-c6d3-461f-9717-3c81fce4740e\"},{\"content\":{\"side\":\"TOP\"},\"type\":\"ConnectorPlacement.EquallySpacedRectSide\",\"uuid\":\"23e2f61e-2083-47d3-9d3a-aca5cd4f1fc6\"}]},\"type\":\"ConnectorPlacement.EquallySpacedConnector\",\"uuid\":\"a2e9d942-417e-49d1-8834-66036fdf29fe\"}],\"packageUris\":[\"http://schema.mathworks.com/mf0/Connector/R2020b\"],\"version\":\"1.0\"}"
  Bus Element Out1 : Outport  PortName=InspT
  wires:
  Bus Element In2/1 -> Heated_Wire/1(HeaterT)
  Bus Element In1/1 -> Heated_Wire/2(HeaterH)
  Heated_Wire/1(InspT) -> Bus Element Out1/1
  Bus Element In4/1 -> Component/1(HumidT)
  Component/1(waterT) -> Temp_RH_Sensor/1(waterT)

== system Logical_Ventilation/Ventilator/Expiratory_System/Expiratory_Tube/CheckValve ==

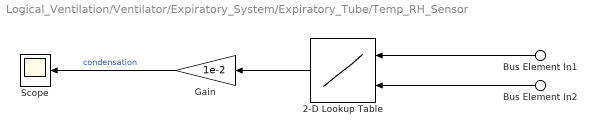
== system Logical_Ventilation/Ventilator/Expiratory_System/Expiratory_Tube/Temp_RH_Sensor ==
  Bus Element In1 : Inport  PortName=ExpSens_T  Element=Water_T
  Bus Element In2 : Inport  PortName=ExpSens_T  Element=heatedWire_T
  2-D Lookup Table : Lookup_n-D  BreakpointsForDimension1=[20 40 45]  BreakpointsForDimension2=[30;37]  Table=[1.75 2.5;2.2 3.1;2.5 3.5]  InternalRulePriority=Speed  RndMeth=Simplest
      settings: InputPortMap=u0,u1
  Gain : Gain  Gain=1e-2
  Scope : Scope
  wires:
  2-D Lookup Table/1 -> Gain/1
  Gain/1 -> Scope/1  "condensation"
  Bus Element In1/1 -> 2-D Lookup Table/1
  Bus Element In2/1 -> 2-D Lookup Table/2

== system Logical_Ventilation/Ventilator/Inspiratory_System/Inspiratory_Tube/CheckValve ==

== system Logical_Ventilation/Ventilator/Inspiratory_System/Inspiratory_Tube/Component ==
  In Bus Element : Inport  PortName=HumidT  Element=Water_T
  Out Bus Element : Outport  PortName=waterT  Element=Water_T
  wires:
  In Bus Element/1 -> Out Bus Element/1

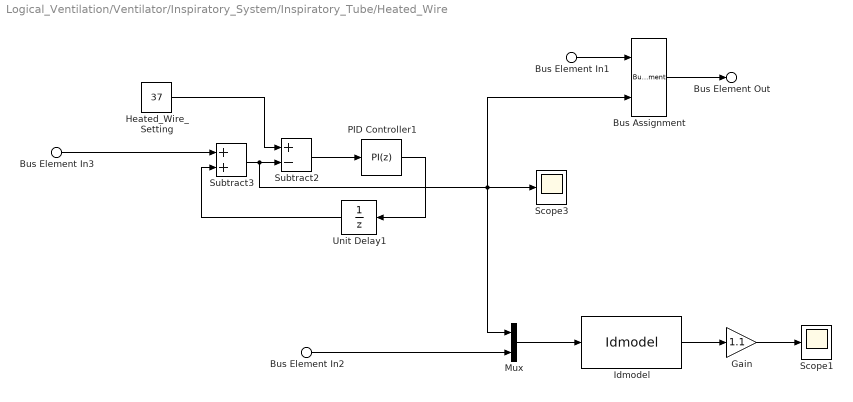
== system Logical_Ventilation/Ventilator/Inspiratory_System/Inspiratory_Tube/Heated_Wire ==
  Bus Element In1 : Inport  PortName=HeaterT
  Bus Element In3 : Inport  PortName=HeaterT  Element=Water_T
  Bus Element In2 : Inport  Port=2  PortName=HeaterH  Element=Humidifier_H
  Bus Assignment : BusAssignment  AssignedSignals=heatedWire_T
  Gain : Gain  Gain=1.1
  Heated_Wire_Setting : Constant  Value=37
  Idmodel : slident/Models/Idmodel  sys=mp_heatedwire  IC=0  noi=on  seed=[]
  Mux : Mux  Inputs=2
  PID Controller1 : slpidlib/PID Controller  Controller=PI  Form=Parallel  TimeDomain=Discrete-time  UseExternalTs=off  SampleTime=0.05  IntegratorMethod=Forward Euler  FilterMethod=Forward Euler  ControllerParametersSource=internal  P=0.0103828718955391  I=0.415314875821562  UseKiTs=off  D=0  N=100  UseFilter=on  TunerSelectOption=Transfer Function Based (PID Tuner App)  InitialConditionSource=internal  InitialConditionForIntegrator=0  InitialConditionForFilter=0  DifferentiatorICPrevScaledInput=0  ExternalReset=none  TrackingMode=off  Kt=1  LimitOutput=off  SatLimitsSource=internal  UpperSaturationLimit=inf  LowerSaturationLimit=-inf  LinearizeAsGain=on  AntiWindupMode=none  Kb=1  LimitIntegrator=off  UpperIntegratorSaturationLimit=inf  LowerIntegratorSaturationLimit=-inf  POutMin=[]  POutMax=[]  IOutMin=[]  IOutMax=[]  DOutMin=[]  DOutMax=[]  NOutMin=[]  NOutMax=[]  SumOutMin=[]  SumOutMax=[]  SaturationOutMin=[]  SaturationOutMax=[]  PParamMin=[]  PParamMax=[]  IParamMin=[]  IParamMax=[]  DParamMin=[]  DParamMax=[]  NParamMin=[]  NParamMax=[]  KbParamMin=[]  KbParamMax=[]  KtParamMin=[]  KtParamMax=[]  KbOutMin=[]  KbOutMax=[]  KtOutMin=[]  KtOutMax=[]  IntegratorOutMin=[]  IntegratorOutMax=[]  FilterOutMin=[]  FilterOutMax=[]  SumI1OutMin=[]  SumI1OutMax=[]  SumI2OutMin=[]  SumI2OutMax=[]  SumI3OutMin=[]  SumI3OutMax=[]  SumI4OutMin=[]  SumI4OutMax=[]  SumDOutMin=[]  SumDOutMax=[]  DifferentiatorOutMin=[]  DifferentiatorOutMax=[]  FilterDiffOutCoefMin=[]  FilterDiffOutCoefMax=[]  ReciprocalOutMin=[]  ReciprocalOutMax=[]  SumDenOutMin=[]  SumDenOutMax=[]  SumNumOutMin=[]  SumNumOutMax=[]  DivideOutMin=[]  DivideOutMax=[]  UdiffTsProdOutMin=[]  UdiffTsProdOutMax=[]  NTsProdOutMin=[]  NTsProdOutMax=[]  UintegralTsProdOutMin=[]  UintegralTsProdOutMax=[]  UngainTsProdOutMin=[]  UngainTsProdOutMax=[]  ClampingZeroOutDataTypeStr=Inherit: Inherit via back propagation  ClampingZeroOutMin=[]  ClampingZeroOutMax=[]  FilterDenConstantOutDataTypeStr=Inherit: Inherit via back propagation  FilterDenConstantOutMin=[]  FilterDenConstantOutMax=[]  PCopyOutDataTypeStr=Inherit: Inherit via back propagation  PCopyOutMin=[]  PCopyOutMax=[]  NCopyOutDataTypeStr=Inherit: Inherit via back propagation  NCopyOutMin=[]  NCopyOutMax=[]  IntegratorContinuousStateAttributes=''  IntegratorStateMustResolveToSignalObject=off  IntegratorRTWStateStorageClass=Auto  FilterContinuousStateAttributes=''  FilterStateMustResolveToSignalObject=off  FilterRTWStateStorageClass=Auto  ParallelPVariant=InternalParameters  IdealPVariant=Disabled  IVariant=InternalParameters  DVariant=Disabled  IntegratorVariant=Discrete  SatVariant=Disabled  AWVariant=Passthrough  PCopyVariant=Disabled  TRVariant=Disabled  FdbkBlocksVariant=Forward  IdealPFdbkVariant=Disabled  SatFdbkVariant=Disabled  DerivativeFilterVariant=Disabled  NVariant=Disabled  NCopyVariant=Disabled_SignalSpec  FilterICVariant=Disabled  IntegratorICVariant=InternalICs  ExternalResetVariant=Disabled  TRSumVariant=Passthrough  SumFdbkVariant=Disabled  SumVariant=Sum_PI  TsampFilterVariant=InternalTs  TsampNgainVariant=Passthrough  TsampIntegralVariant=Disabled_SignalSpec  ExternalSaturationOutDataTypeStr=Inherit: Same as second input
  Scope1 : Scope
  Scope3 : Scope
  Subtract2 : Sum  Inputs=+-
  Subtract3 : Sum
  Unit Delay1 : UnitDelay  SampleTime=-1  HasFrameUpgradeWarning=on
  Bus Element Out : Outport  PortName=InspT
  wires:
  PID Controller1/1 -> Unit Delay1/1
  Bus Element In3/1 -> Subtract3/1
  Unit Delay1/1 -> Subtract3/2
  Subtract3/1 -> Mux/1, Bus Assignment/2, Scope3/1, Subtract2/2
  Subtract2/1 -> PID Controller1/1
  Heated_Wire_Setting/1 -> Subtract2/1
  Mux/1 -> Idmodel/1
  Idmodel/1 -> Gain/1
  Gain/1 -> Scope1/1
  Bus Element In2/1 -> Mux/2
  Bus Element In1/1 -> Bus Assignment/1
  Bus Assignment/1 -> Bus Element Out/1

== system Logical_Ventilation/Ventilator/Inspiratory_System/Inspiratory_Tube/Temp_RH_Sensor ==
  Bus Element In1 : Inport  PortName=waterT
  1-D Lookup Table : Lookup_n-D  NumberOfTableDimensions=1  BreakpointsForDimension1=[20 25 30 35 40 45]  Table=[0.25 0.3 0.375 0.475 0.6 0.7]  InternalRulePriority=Speed  RndMeth=Simplest
  Scope : Scope
  Bus Element Out : Outport  PortName=SensH  Element=Insp_Humidity
  wires:
  1-D Lookup Table/1 -> Bus Element Out/1, Scope/1  "Inspiration_Humidity"
  Bus Element In1/1 -> 1-D Lookup Table/1
